simulink model "three_phase_inverter_step_signal"  (R2025a)
settings: Solver=VariableStepAuto  StartTime=0.0  StopTime=10.0  RelTol=1e-3
libraries: spsVoltageMeasurementLib x6, spsIGBTLib x6, spsCurrentMeasurementLib x3, spsSeriesRLCLoadLib x3, spsDCVoltageSourceLib x1, sps_lib x1
settings Model: Creator=ayush  LastModifiedBy=ayush

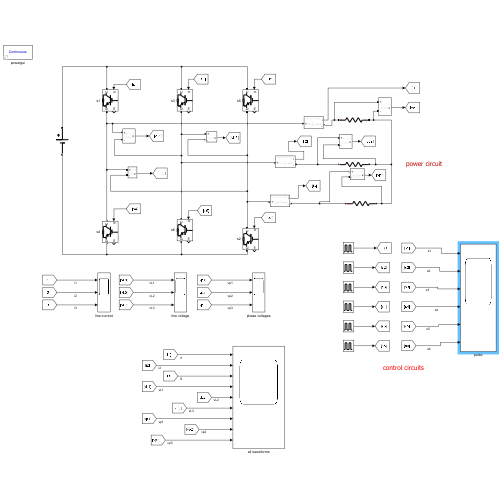
[thumbnail: Simulink's stored preview of the top-level diagram]
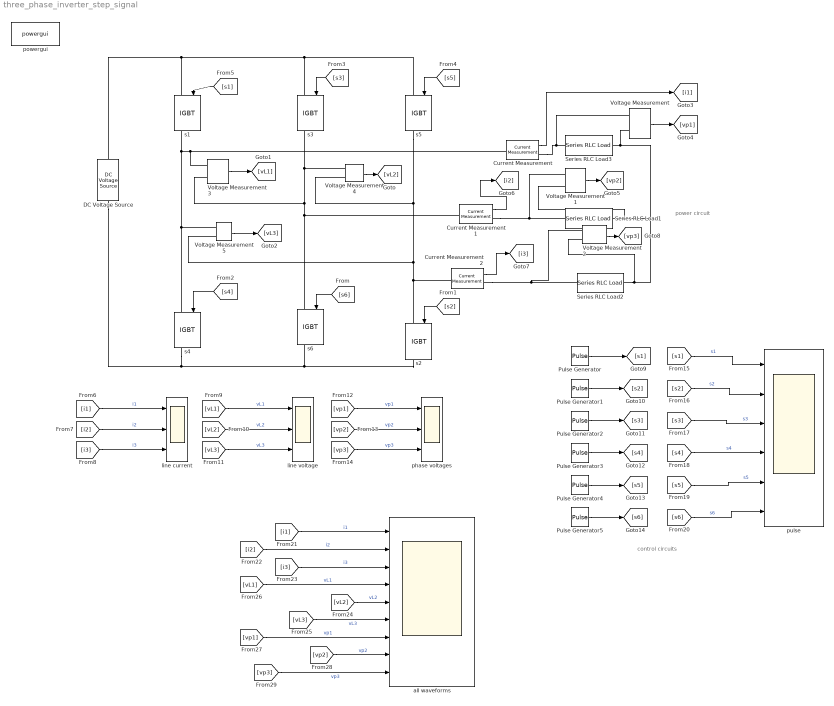
== system three_phase_inverter_step_signal ==
  note: control circuits
  note: power circuit
  Current Measurement : spsCurrentMeasurementLib/Current Measurement  PhasorSimulation=off  OutputType=Complex  PSBequivalent=0
  Current Measurement1 : spsCurrentMeasurementLib/Current Measurement  PhasorSimulation=off  OutputType=Complex  PSBequivalent=0
  Current Measurement2 : spsCurrentMeasurementLib/Current Measurement  PhasorSimulation=off  OutputType=Complex  PSBequivalent=0
  DC Voltage Source : spsDCVoltageSourceLib/DC Voltage Source  Amplitude=50  Measurements=None
  Pulse Generator : DiscretePulseGenerator  PulseType=Time based  Period=0.02  PulseWidth=50
  Pulse Generator1 : DiscretePulseGenerator  PulseType=Time based  Period=0.02  PulseWidth=50  PhaseDelay=60*0.02/360
  Pulse Generator2 : DiscretePulseGenerator  PulseType=Time based  Period=0.02  PulseWidth=50  PhaseDelay=120*0.02/360
  Pulse Generator3 : DiscretePulseGenerator  PulseType=Time based  Period=0.02  PulseWidth=50  PhaseDelay=180*0.02/360
  Pulse Generator4 : DiscretePulseGenerator  PulseType=Time based  Period=0.02  PulseWidth=50  PhaseDelay=240*0.02/360
  Pulse Generator5 : DiscretePulseGenerator  PulseType=Time based  Period=0.02  PulseWidth=50  PhaseDelay=300*0.02/360
  Series RLC Load1 : spsSeriesRLCLoadLib/Series RLC Load  LConnTagsString=a  RConnTagsString=__new0  NominalVoltage=1000  NominalFrequency=60  ActivePower=10e3  InductivePower=0  CapacitivePower=0  Setx0=off  InitialVoltage=0  SetiL0=off  InitialCurrent=0  Measurements=None  LoadType=constant Z
  Series RLC Load2 : spsSeriesRLCLoadLib/Series RLC Load  LConnTagsString=a  RConnTagsString=__new0  NominalVoltage=1000  NominalFrequency=60  ActivePower=10e3  InductivePower=0  CapacitivePower=0  Setx0=off  InitialVoltage=0  SetiL0=off  InitialCurrent=0  Measurements=None  LoadType=constant Z
  Series RLC Load3 : spsSeriesRLCLoadLib/Series RLC Load  LConnTagsString=a  RConnTagsString=__new0  NominalVoltage=1000  NominalFrequency=60  ActivePower=10e3  InductivePower=0  CapacitivePower=0  Setx0=off  InitialVoltage=0  SetiL0=off  InitialCurrent=0  Measurements=None  LoadType=constant Z
  Voltage Measurement{,1..5} (6 alike) : spsVoltageMeasurementLib/Voltage Measurement  PhasorSimulation=off  OutputType=Complex  PSBequivalent=0
  all waveforms : Scope  NumInputPorts=9
      settings: ActiveDisplayYMinimum=-0.39999599204015984  ActiveDisplayYMaximum=0.39999599204015979  DataLoggingVariableName=ScopeData4
  line current : Scope  NumInputPorts=3
      settings: ActiveDisplayYMinimum=-0.39999599204015984  ActiveDisplayYMaximum=0.39999599204015984
  line voltage : Scope  NumInputPorts=3
      settings: ActiveDisplayYMinimum=-59.999398806023969  ActiveDisplayYMaximum=59.999398806023969
  phase voltages : Scope  NumInputPorts=3
      settings: ActiveDisplayYMinimum=-39.999599204015972  ActiveDisplayYMaximum=39.999599204015979  DataLoggingVariableName=ScopeData2
  powergui : sps_lib/powergui  Priority=1  SimulationMode=Continuous  SampleTime=50e-6  frequency=60  Iterations=50  frequencyindice=0  Pbase=100e6  ErrMax=1e-4  UnitsV=kV  UnitsW=MW  buscounter=0  FunctionMessages=off  echomessages=off  EnableUseOfTLC=off  CurrentSourceSwitches=off  DisableSnubberDevices=off  DisableRonSwitches=off  DisableVfSwitches=off  DisplayEquations=off  AutomaticDiscreteSolvers=off  SolverType=Tustin/Backward Euler (TBE)  Interpol=off  ExternalGateDelay=off  methode=off  Ts=100  x0status=blocks  SPID=on  SwTol=0  HookPort=off  NonlinearTolerance=1e-4  nMaxIteration=100  ContinueOnMaxIteration=off  RestoreLinks=warning  ResistiveCurrentMeasurement=off  Frange=[0:2:500]  Ylog=off  Xlog=on  ShowGrid=off  save=off  variable=ZData  structure=0  ZoomFFT=off  StartTime=0.0  cycles=1  DisplayStyle=1  fundamental=60  FreqAxis=off  MaxFrequency=1000  frequencyindicesteady=1  RmsSteady=1  display=off
  pulse : Scope  NumInputPorts=6
      settings: ActiveDisplayYMinimum=-0.12499999999999997  ActiveDisplayYMaximum=1.125  DataLoggingVariableName=ScopeData3
  s{1..6} (6 alike) : spsIGBTLib/IGBT  Ron=0.001  Lon=0  Vf=1  Tf=1e-6  Tt=2e-6  IC=0  Rs=1e5  Cs=inf  Measurements=on
  wires:
  Current Measurement/1 -> [i1]
  [s1] -> s1/1
  [s5] -> s5/1
  [s2] -> s2/1
  [s6] -> s6/1
  [s4] -> s4/1
  Voltage Measurement2/1 -> [vp3]
  Current Measurement2/1 -> [i3]
  Current Measurement1/1 -> [i2]
  Voltage Measurement1/1 -> [vp2]
  Voltage Measurement/1 -> [vp1]
  [i1] -> line current/1  "i1"
  [i2] -> line current/2  "i2"
  [i3] -> line current/3  "i3"
  [vL1] -> line voltage/1  "vL1"
  [vL2] -> line voltage/2  "vL2"
  [vL3] -> line voltage/3  "vL3"
  [vp1] -> phase voltages/1  "vp1"
  [vp2] -> phase voltages/2  "vp2"
  [vp3] -> phase voltages/3  "vp3"
  Voltage Measurement3/1 -> [vL1]
  Voltage Measurement4/1 -> [vL2]
  Voltage Measurement5/1 -> [vL3]
  Pulse Generator/1 -> [s1]
  Pulse Generator1/1 -> [s2]
  Pulse Generator2/1 -> [s3]
  Pulse Generator3/1 -> [s4]
  Pulse Generator4/1 -> [s5]
  Pulse Generator5/1 -> [s6]
  [s3] -> s3/1
  [s1] -> pulse/1  "s1"
  [s2] -> pulse/2  "s2"
  [s3] -> pulse/3  "s3"
  [s4] -> pulse/4  "s4"
  [s5] -> pulse/5  "s5"
  [s6] -> pulse/6  "s6"
  [i1] -> all waveforms/1  "i1"
  [i2] -> all waveforms/2  "i2"
  [i3] -> all waveforms/3  "i3"
  [vL1] -> all waveforms/4  "vL1"
  [vL2] -> all waveforms/5  "vL2"
  [vL3] -> all waveforms/6  "vL3"
  [vp1] -> all waveforms/7  "vp1"
  [vp2] -> all waveforms/8  "vp2"
  [vp3] -> all waveforms/9  "vp3"
  connections:
  s5/RConn1 -- s2/LConn1 -- Current Measurement2/LConn1 -- Voltage Measurement5/LConn2 -- Voltage Measurement4/LConn2
  s2/RConn1 -- DC Voltage Source/LConn1 -- s4/RConn1 -- s6/RConn1
  s6/LConn1 -- Current Measurement1/LConn1 -- Voltage Measurement3/LConn2 -- Voltage Measurement4/LConn1 -- s3/RConn1
  s4/LConn1 -- Current Measurement/LConn1 -- Voltage Measurement3/LConn1 -- s1/RConn1 -- Voltage Measurement5/LConn1
  s1/LConn1 -- s5/LConn1 -- s3/LConn1 -- DC Voltage Source/RConn1
  Series RLC Load2/RConn1 -- Voltage Measurement2/LConn2 -- Voltage Measurement/LConn2 -- Series RLC Load3/RConn1 -- Voltage Measurement1/LConn2 -- Series RLC Load1/RConn1
  Current Measurement/RConn1 -- Voltage Measurement/LConn1 -- Series RLC Load3/LConn1
  Current Measurement2/RConn1 -- Voltage Measurement2/LConn1 -- Series RLC Load2/LConn1
  Current Measurement1/RConn1 -- Voltage Measurement1/LConn1 -- Series RLC Load1/LConn1
